simulink model "rover_2d_suspension2_motors"  (R2021a)
settings: Solver=ode23t  StartTime=0.0  StopTime=160  RelTol=1e-3
values from neighbouring files (symbols this model uses):
  s = tf('s')    [Apollo_LM_design_discrete_observer.m]    (also in elastic_shaft_rlocus.m; harmonic_osc_rlocus.m)
undefined symbols (not defined in the file or in its folder): X, Y, Z
libraries: sm_lib x77, nesl_utility x18
(part 1 of 2)
settings Model: Creator=kjartan  LastModifiedBy=kjartan

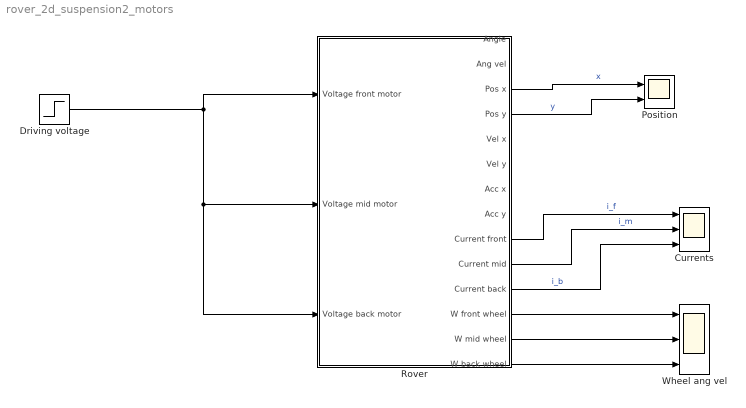
== system rover_2d_suspension2_motors ==
  Currents : Scope  NumInputPorts=3
  Driving voltage : Step  Time=5  After=48  SampleTime=0
  Position : Scope  NumInputPorts=2
  Rover : Subsystem
  Wheel ang vel : Scope  NumInputPorts=3
  wires:
  Driving voltage/1 -> Rover/3(Voltage back motor), Rover/2(Voltage mid motor), Rover/1(Voltage front motor)
  Rover/3(Pos x) -> Position/1  "x"
  Rover/9(Current front) -> Currents/1  "i_f"
  Rover/10(Current mid) -> Currents/2  "i_m"
  Rover/11(Current back) -> Currents/3  "i_b"
  Rover/4(Pos y) -> Position/2  "y"
  Rover/12(W front wheel) -> Wheel ang vel/1
  Rover/13(W mid wheel) -> Wheel ang vel/2
  Rover/14(W back wheel) -> Wheel ang vel/3
